simulink model "freeze_cntr_test"  (Simulink 7.0)
settings: Solver=VariableStepDiscrete  StartTime=0.0  StopTime=1000  RelTol=1e-3
libraries: xbsIndex_r4 x8, casper_library x1
settings Model: Creator=User  LastModifiedBy=User
settings DebuggingCC: SaveWithDisabledLinksMsg=none  SaveWithParameterizedLinksMsg=none

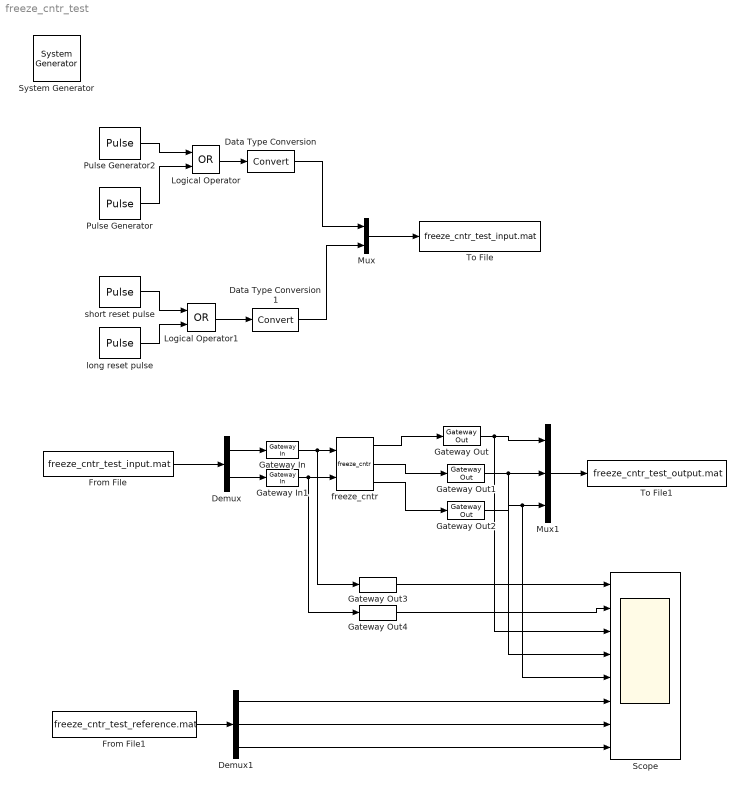
== system freeze_cntr_test ==
  " System Generator" : xbsIndex_r4/ System Generator  Tag=genX  SystemSampleTime=-1  xilinxfamily=Virtex4  part=xc4vsx35  speed=-10  package=ff668  synthesis_tool=XST  clock_wrapper=Clock Enables  directory=./netlist  testbench=off  simulink_period=1  sysclk_period=100  dcm_input_clock_period=100  incr_netlist=off  trim_vbits=Everywhere in SubSystem  dbl_ovrd=According to Block Masks  core_generation=According to Block Masks  run_coregen=off  deprecated_control=off  eval_field=0  block_type=sysgen
      settings: block_version=10.1.1
  Data Type Conversion : DataTypeConversion  OutDataTypeMode=double  OutDataType=sfix(16)  OutScaling=2^0
  Data Type Conversion1 : DataTypeConversion  OutDataTypeMode=double  OutDataType=sfix(16)  OutScaling=2^0
  Demux : Demux  Outputs=2
  Demux1 : Demux  Outputs=3
  From File : FromFile  FileName=freeze_cntr_test_input.mat  SampleTime=1
  From File1 : FromFile  FileName=freeze_cntr_test_reference.mat  SampleTime=1
  Gateway In : xbsIndex_r4/Gateway In  arith_type=Boolean  n_bits=16  bin_pt=14  quantization="Round  (unbiased: +/- Inf)"  overflow=Saturate  period=1  dbl_ovrd=off  timing_constraint=None  locs_specified=off  LOCs={}  block_type=gatewayin
      settings: infoedit="Gateway in block.  Converts inputs of type Simulink integer, double and fixed point to  Xilinx fixed point type.<P><P>Hardware notes:  In hardware these blocks become top level input ports."  block_version=10.1.1
  Gateway In1 : xbsIndex_r4/Gateway In  arith_type=Boolean  n_bits=16  bin_pt=14  quantization="Round  (unbiased: +/- Inf)"  overflow=Saturate  period=1  dbl_ovrd=off  timing_constraint=None  locs_specified=off  LOCs={}  block_type=gatewayin
      settings: infoedit="Gateway in block.  Converts inputs of type Simulink integer, double and fixed point to  Xilinx fixed point type.<P><P>Hardware notes:  In hardware these blocks become top level input ports."  block_version=10.1.1
  Gateway Out{,1..4} (5 alike) : xbsIndex_r4/Gateway Out  hdl_port=on  timing_constraint=None  locs_specified=off  LOCs={}  block_type=gatewayout
      settings: infoedit="Gateway out block.  Converts Xilinx fixed point inputs into ouputs of type Simulink integer, double, or fixed point.<P><P>Hardware notes:  In hardware these blocks become top level output ports or are discarded, depending on how they are configured."  block_version=10.1.1
  Logical Operator : Logic  Operator=OR  AllPortsSameDT=off  OutDataTypeMode=boolean
  Logical Operator1 : Logic  Operator=OR  AllPortsSameDT=off  OutDataTypeMode=boolean
  Mux : Mux  Inputs=2
  Mux1 : Mux  Inputs=3
  Pulse Generator : DiscretePulseGenerator  Period=30  PulseWidth=15  PhaseDelay=10
  Pulse Generator2 : DiscretePulseGenerator  Period=50  PulseWidth=30  PhaseDelay=20
  Scope : Scope  NumInputPorts=8
      settings: YMin=-5~-5~-5~-5~-5~-5~-5~-5  YMax=5~5~5~5~5~5~5~5
  To File : ToFile  Filename=freeze_cntr_test_input.mat  MatrixName=input
  To File1 : ToFile  Filename=freeze_cntr_test_output.mat  MatrixName=output
  freeze_cntr : casper_library/Misc/freeze_cntr  SystemSampleTime=-1  CounterBits=6
  long reset pulse : DiscretePulseGenerator  Period=221  PulseWidth=4  PhaseDelay=5
  short reset pulse : DiscretePulseGenerator  Period=150  PhaseDelay=5
  wires:
  short reset pulse/1 -> Logical Operator1/1
  long reset pulse/1 -> Logical Operator1/2
  Pulse Generator2/1 -> Logical Operator/1
  Pulse Generator/1 -> Logical Operator/2
  Logical Operator/1 -> Data Type Conversion/1
  Logical Operator1/1 -> Data Type Conversion1/1
  Data Type Conversion/1 -> Mux/1
  Data Type Conversion1/1 -> Mux/2
  Mux/1 -> To File/1
  From File/1 -> Demux/1
  Demux/1 -> Gateway In/1
  Demux/2 -> Gateway In1/1
  Gateway In/1 -> freeze_cntr/1, Gateway Out3/1
  Gateway In1/1 -> freeze_cntr/2, Gateway Out4/1
  freeze_cntr/1 -> Gateway Out/1
  freeze_cntr/2 -> Gateway Out1/1
  freeze_cntr/3 -> Gateway Out2/1
  Gateway Out/1 -> Mux1/1, Scope/3
  Gateway Out1/1 -> Mux1/2, Scope/4
  Gateway Out2/1 -> Mux1/3, Scope/5
  Mux1/1 -> To File1/1
  Gateway Out3/1 -> Scope/1
  Gateway Out4/1 -> Scope/2
  From File1/1 -> Demux1/1
  Demux1/1 -> Scope/6
  Demux1/2 -> Scope/7
  Demux1/3 -> Scope/8
